simulink model "esp_func"  (R2020b)
settings: Solver=ode23t  StartTime=0.0  StopTime=Tf  RelTol=1e-2
model workspace: external: MAT-File C:\PhD\Variable Threshold\demo_rl.mat (data not in the file)
values from neighbouring files (symbols this model uses):
  Tf = 200    [RLenv.m]    (also in RlEnvModel.m; demo_rl.m; main_rl.m = simlen*Ts; main_rl_func_modified.m = simlen*Ts)
  Ts = 0.1    [RLenv.m]    (also in RlEnvModel.m; demo_rl.m; main_rl.m = s.Ts; main_rl_func_modified.m = s.Ts)
libraries: simulink x2
settings Model: Creator=The MathWorks, Inc.  LastModifiedBy=IIT_KGP_CSE_FM_LAB

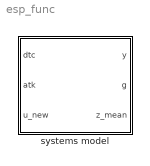
== system esp_func ==
  systems model : Subsystem

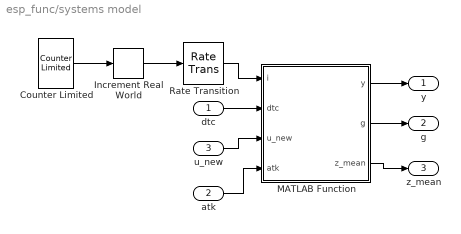
== system esp_func/systems model ==
  dtc : Inport
  atk : Inport  Port=2
  u_new : Inport  Port=3
  Counter Limited : simulink/Sources/Counter Limited  uplimit=Tf/Ts  tsamp=Ts
  Increment Real World : simulink/Additional Math & Discrete/Additional Math: Increment - Decrement/Increment Real World
      settings: SourceProductBaseCode=SL
  MATLAB Function : MATLAB Function  TreatAsAtomicUnit=on
  Rate Transition : RateTransition
  y : Outport
  g : Outport  Port=2
  z_mean : Outport  Port=3
  wires:
  MATLAB Function/3(z_mean) -> z_mean/1
  MATLAB Function/2(g) -> g/1
  Increment Real World/1 -> Rate Transition/1
  MATLAB Function/1(y) -> y/1
  atk/1 -> MATLAB Function/4(atk)
  Rate Transition/1 -> MATLAB Function/1(i)
  Counter Limited/1 -> Increment Real World/1
  dtc/1 -> MATLAB Function/2(dtc)
  u_new/1 -> MATLAB Function/3(u_new)

== matlab function esp_func/systems model/MATLAB Function ==
  data: i input; y output; g output; z_mean output; dtc input; u_new input; atk input; s parameter
function [y,g,z_mean] = env(i,dtc,u_new,atk, s)
% function [y,g,z_mean]= envSys(atk,dtc,new_u,ref, s)
%% SYS_ENV Summary of this function goes here

%%%%%%%%%%%%%%%%%%%%%%%%%%%=====FDI Attack=========%%%%%%%%%%%%%%%%%%%%%
%========================== obtained from code ======================%
% x1_0=-15.0;
% x2_0=16.6096079397;
% fdi_u=[ 35.99313719  71.98627437  58.33575204  41.29588025   0.   0.         -31.21892088  -5.09118639   0.           0.  -0.41831677   0.           0.           0.           0.   0. ];
% fdi_y=[15.01515367 13.48175215 11.26355514 10.30553807  8.22658704  4.85366237  3.61911687  2.21566942  1.21608204  0.53164255  0.1748743   0.  0.          0.          0.          0. ];
%======================================================================%

% ay=  [fdi_y,zeros(1,time-size(fdi_y,2))];
% au = [fdi_u,zeros(1,time-size(fdi_u,2))];

%%%%%%%%%%%%%%%%%%%%%%%%%%=====System Simulation======%%%%%%%%%%%%%%%%%%

%====================Chi Squared Test =================
% tau = 1; % Detection window % new: let's check for every iteration now
%======================================================
% stateProg(esp_env,i,dtc(2),dtc(1),new_u,atk(1),atk(2))
au= atk(1);

ay= atk(2);
th= dtc(1);
tau= dtc(2);
% coder.extrinsic('evalin','assignin');
% evalin
%  for i = 1:esp_env.Ts:esp_env.Tf
    
    
            s.t(i+1)=i*s.Ts;
            s.a_u(:,i+1)=au;
            s.a_y(:,i+1)=ay;
            s.x_act(:,i+1) = s.A*s.x_act(i)+s.B*s.uatk(i)+s.proc_noise(i);
%             s.xatk(i)= s.A*s.x_act(i)+s.B*s.u_act(i);
            s.xhat(:,i+1) = s.A*s.xhat(i) + s.B*s.u_act(i) + s.L*s.z(i);
            s.est_err(:,i+1)= s.x_act(:,i+1)-s.xhat(:,i+1);
            s.u_act(:,i+1)= s.K*s.xhat(:,i+1);
            s.uatk(:,i+1)= s.u_act(:,i+1)+s.a_u(:,i+1);
            s.y_act(:,i+1)= s.C*s.x_act(i+1)+s.meas_noise(i);
            s.yatk(:,i+1)= s.y_act(:,i+1)+s.a_y(:,i+1);
            s.z(:,i+1)= s.yatk(:,i+1)-C*s.xhat(:,i+1);
            s.z_mean(:,i+1)= mean(s.z);
            s.P = cov(s.z');
            s.chi_tst(i+1)= z(:,i+1)'*inv(P)*z(:,i+1);
            s.threshold(i+1)= th;
            s.tau(i+1)= dtc_windw;
            s.g(i+1) = 0;               
%             if i-tau+1 > 0                  % Calculate detector window starting index
%                 srt = i-tau+1;              % tau is the detector window length
%             else
%                 srt = 1;
%             end
            for k = max(1,i-s.tau(i+1)+1):i+1
                s.g(i+1) = s.g(i+1) + s.chi_tst(k);  % Calculate gk (chi2 test)
            end
            if s.g(i+1) > s.threshold(i+1)
                s.u_act(:,i+1) = u_new;
                s.uatk(:,i+1)= s.u_act(:,i+1)+s.a_u(:,i+1);
                isatk=1;
            else
                isatk=0;
            end

    g= s.g(i+1);
    y=s.yatk(:,i+1);
    z_mean = s.z_mean(i+1);

end
